simulink model "multi_UAV_simulation_model"  (R2023b)
settings: Solver=FixedStepAuto  StartTime=0  StopTime=end_time  FixedStep=0.01  RelTol=1e-3
values from neighbouring files (symbols this model uses):
  M_gamma = double(M_gamma)    [variable_system.m]
undefined symbols (not defined in the file or in its folder): AX_all, AY_all, F_dist, f_max, gamma0, J, J_xi, m, opt_angle_table_mat, tau_rotor, x0
libraries: slpidlib x4
settings Model: Creator=mochida  LastModifiedBy=tito
settings SolverCC: AlgebraicLoopSolver=TrustRegion
settings DataIOCC: SaveFormat=StructureWithTime  ReturnWorkspaceOutputs=off
settings OptimizationCC: BlockReduction=off  BufferReuse=off
settings DebuggingCC: AlgebraicLoopMsg=none  ArithmeticOperatorsInVariantConditions=warning
settings ModelReferenceCC: EnableRefExpFcnMdlSchedulingChecks=on
settings SFSimCC: SimUseLocalCustomCode=off  CustomCodeUndefinedFunction=UseInterfaceOnly
settings RTWCC: RTWUseLocalCustomCode=off  DLArmComputeVersion=19.05
settings ExplorerConfigSet: SimMechanicsOpenEditorOnUpdate=off

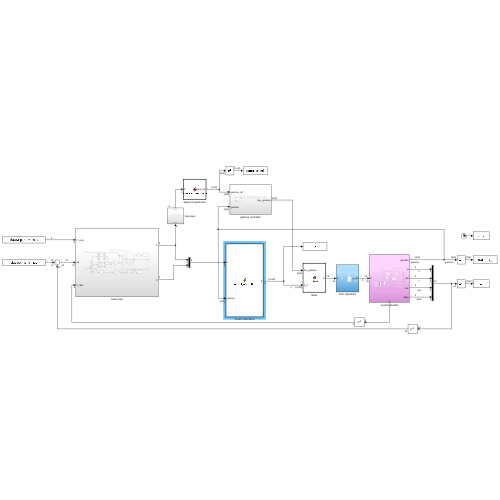
[thumbnail: Simulink's stored preview of the top-level diagram]
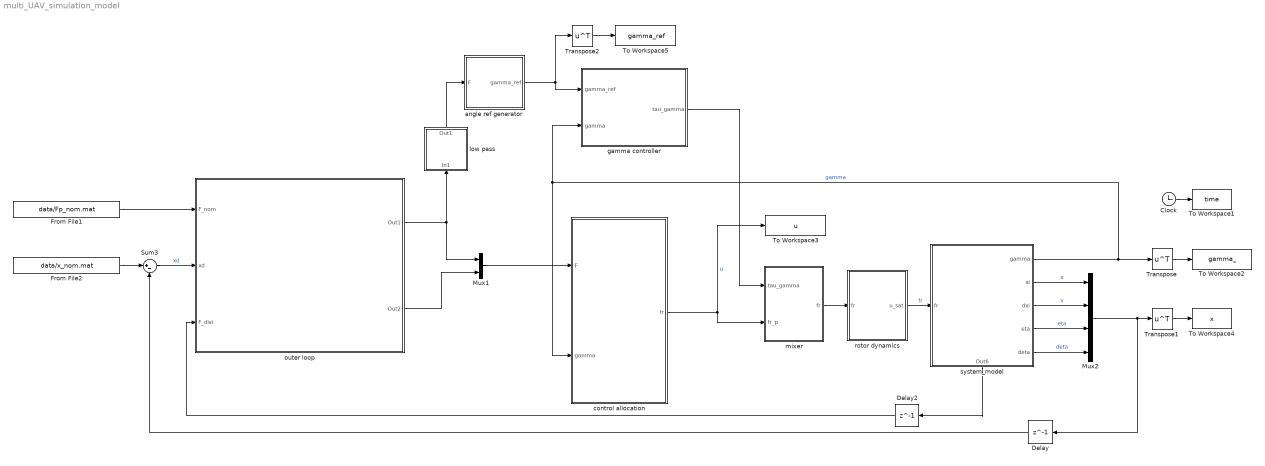
== system multi_UAV_simulation_model ==
  Clock : Clock
  Delay : Delay  DelayLength=1  InitialCondition=x0
  Delay2 : Delay  DelayLength=1  InitialCondition=zeros(3,1)
  From File1 : FromFile  FileName=data/Fp_nom.mat  SampleTime=0  ExtrapolationAfterLastDataPoint=Hold last value
  From File2 : FromFile  FileName=data/x_nom.mat  SampleTime=0  ExtrapolationAfterLastDataPoint=Hold last value
  Mux1 : Mux  Inputs=2
  Mux2 : Mux
  Sum3 : Sum  Inputs=|+-
  To Workspace1 : ToWorkspace  VariableName=time  SampleTime=-1
  To Workspace2 : ToWorkspace  VariableName=gamma_  SampleTime=-1
      settings: Save2DSignal=2-D array (concatenate along first dimension)
  To Workspace3 : ToWorkspace  VariableName=u  SampleTime=-1
  To Workspace4 : ToWorkspace  VariableName=x  SampleTime=-1
      settings: Save2DSignal=2-D array (concatenate along first dimension)
  To Workspace5 : ToWorkspace  VariableName=gamma_ref  SampleTime=-1
      settings: Save2DSignal=2-D array (concatenate along first dimension)
  Transpose : Math  Operator=transpose
  Transpose1 : Math  Operator=transpose
  Transpose2 : Math  Operator=transpose
  angle ref generator : MATLAB Function  TreatAsAtomicUnit=on
  control allocation : MATLAB Function  TreatAsAtomicUnit=on
  gamma controller : Subsystem
  low pass : Subsystem
  mixer : MATLAB Function  TreatAsAtomicUnit=on
  outer loop : Subsystem
  rotor dynamics : Subsystem
  system_model : Subsystem
      settings: PortSchema="{\"entries\":[{\"content\":{\"sides\":[{\"content\":{\"connectorIds\":[\"In1\"]},\"type\":\"ConnectorPlacement.EquallySpacedRectSide\",\"uuid\":\"254c1886-4b3f-4fd7-a815-da90215f9171\"},{\"content\":{\"connectorIds\":[\"Out1\",\"Out2\",\"Out3\",\"Out4\",\"Out5\"],\"side\":\"RIGHT\"},\"type\":\"ConnectorPlacement.EquallySpacedRectSide\",\"uuid\":\"0b427131-5008-4b05-bf64-69ca1b176e39\"},{\"content\":{\"side\":\"TOP\"},\"type\":\"ConnectorPlacement.EquallySpacedRectSide\",\"uuid\":\"ac393484-bc2a-4ae6-a0d7-f6f44710c509\"},{\"content\":{\"connectorIds\":[\"Out6\"],\"side\":\"BOTTOM\"},\"type\":\"ConnectorPlacement.EquallySpacedRectSide\",\"uuid\":\"d50d45f9-0e3b-4b3e-8f4a-1a82dc9ea554\"}]},\"type\":\"ConnectorPlacement.EquallySpacedConnector\",\"uuid\":\"c72c2ee8-503c-4769-877b-d1646d141d46\"}],\"packageUris\":[\"http://schema.mathworks.com/mf0/Connector/R2020b\"],\"version\":\"1.0\"}"
  wires:
  Clock/1 -> To Workspace1/1
  system_model/2(xi) -> Mux2/1  "x"
  system_model/3(dxi) -> Mux2/2  "v"
  system_model/4(eta) -> Mux2/3  "eta"
  system_model/5(deta) -> Mux2/4  "deta"
  rotor dynamics/1(u_sat) -> system_model/1(fr)  "fr"
  control allocation/1(fr) -> To Workspace3/1, mixer/2(fr_p)  "u"
  Delay/1 -> Sum3/2
  mixer/1(fr) -> rotor dynamics/1(fr)
  From File2/1 -> Sum3/1
  Mux2/1 -> Delay/1, Transpose1/1
  Transpose/1 -> To Workspace2/1
  Transpose1/1 -> To Workspace4/1
  system_model/1(gamma) -> gamma controller/2(gamma), control allocation/2(gamma), Transpose/1  "gamma"
  Mux1/1 -> control allocation/1(F)
  gamma controller/1(tau_gamma) -> mixer/1(tau_gamma)
  low pass/1(Out1) -> angle ref generator/1(F)
  angle ref generator/1(gamma_ref) -> Transpose2/1, gamma controller/1(gamma_ref)
  system_model/6(Out6) -> Delay2/1
  outer loop/1(Out1) -> low pass/1(In1), Mux1/1
  Sum3/1 -> outer loop/2(xd)  "xd"
  Delay2/1 -> outer loop/3(F_dist)
  outer loop/2(Out2) -> Mux1/2
  From File1/1 -> outer loop/1(F_nom)
  Transpose2/1 -> To Workspace5/1

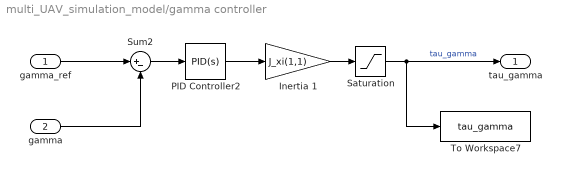
== system multi_UAV_simulation_model/gamma controller ==
  gamma_ref : Inport
  gamma : Inport  Port=2
  Inertia 1 : Gain  Gain=J_xi(1,1)
  PID Controller2 : slpidlib/PID Controller  Controller=PID  Form=Parallel  TimeDomain=Continuous-time  UseExternalTs=off  SampleTime=-1  IntegratorMethod=Forward Euler  FilterMethod=Forward Euler  ControllerParametersSource=internal  P=20  I=1  UseKiTs=off  D=5  N=209.794311620465  UseFilter=on  TunerSelectOption=Transfer Function Based (PID Tuner App)  InitialConditionSource=internal  InitialConditionForIntegrator=0  InitialConditionForFilter=0  DifferentiatorICPrevScaledInput=0  ExternalReset=none  TrackingMode=off  Kt=1  LimitOutput=off  SatLimitsSource=internal  UpperSaturationLimit=inf  LowerSaturationLimit=-inf  LinearizeAsGain=on  AntiWindupMode=none  Kb=1  LimitIntegrator=off  UpperIntegratorSaturationLimit=inf  LowerIntegratorSaturationLimit=-inf  POutMin=[]  POutMax=[]  IOutMin=[]  IOutMax=[]  DOutMin=[]  DOutMax=[]  NOutMin=[]  NOutMax=[]  SumOutMin=[]  SumOutMax=[]  SaturationOutMin=[]  SaturationOutMax=[]  PParamMin=[]  PParamMax=[]  IParamMin=[]  IParamMax=[]  DParamMin=[]  DParamMax=[]  NParamMin=[]  NParamMax=[]  KbParamMin=[]  KbParamMax=[]  KtParamMin=[]  KtParamMax=[]  KbOutMin=[]  KbOutMax=[]  KtOutMin=[]  KtOutMax=[]  IntegratorOutMin=[]  IntegratorOutMax=[]  FilterOutMin=[]  FilterOutMax=[]  SumI1OutMin=[]  SumI1OutMax=[]  SumI2OutMin=[]  SumI2OutMax=[]  SumI3OutMin=[]  SumI3OutMax=[]  SumI4OutMin=[]  SumI4OutMax=[]  SumDOutMin=[]  SumDOutMax=[]  DifferentiatorOutMin=[]  DifferentiatorOutMax=[]  FilterDiffOutCoefMin=[]  FilterDiffOutCoefMax=[]  ReciprocalOutMin=[]  ReciprocalOutMax=[]  SumDenOutMin=[]  SumDenOutMax=[]  SumNumOutMin=[]  SumNumOutMax=[]  DivideOutMin=[]  DivideOutMax=[]  UdiffTsProdOutMin=[]  UdiffTsProdOutMax=[]  NTsProdOutMin=[]  NTsProdOutMax=[]  UintegralTsProdOutMin=[]  UintegralTsProdOutMax=[]  UngainTsProdOutMin=[]  UngainTsProdOutMax=[]  ClampingZeroOutDataTypeStr=Inherit: Inherit via back propagation  ClampingZeroOutMin=[]  ClampingZeroOutMax=[]  FilterDenConstantOutDataTypeStr=Inherit: Inherit via back propagation  FilterDenConstantOutMin=[]  FilterDenConstantOutMax=[]  PCopyOutDataTypeStr=Inherit: Inherit via back propagation  PCopyOutMin=[]  PCopyOutMax=[]  NCopyOutDataTypeStr=Inherit: Inherit via back propagation  NCopyOutMin=[]  NCopyOutMax=[]  IntegratorContinuousStateAttributes=''  IntegratorStateMustResolveToSignalObject=off  IntegratorRTWStateStorageClass=Auto  FilterContinuousStateAttributes=''  FilterStateMustResolveToSignalObject=off  FilterRTWStateStorageClass=Auto  ParallelPVariant=InternalParameters  IdealPVariant=Disabled  IVariant=InternalParameters  DVariant=InternalParameters  IntegratorVariant=Continuous  SatVariant=Disabled  AWVariant=Passthrough  PCopyVariant=Disabled  TRVariant=Disabled  FdbkBlocksVariant=Forward  IdealPFdbkVariant=Disabled  SatFdbkVariant=Disabled  DerivativeFilterVariant=ContFilter  NVariant=InternalParameters  NCopyVariant=Disabled  FilterICVariant=InternalICsFilter  IntegratorICVariant=InternalICs  ExternalResetVariant=Disabled  TRSumVariant=Passthrough  SumFdbkVariant=Disabled  SumVariant=Sum_PID  TsampFilterVariant=InternalTs  TsampNgainVariant=Passthrough  TsampIntegralVariant=Disabled_SignalSpec  ExternalSaturationOutDataTypeStr=Inherit: Same as second input
  Saturation : Saturate  UpperLimit=0.03  LowerLimit=-0.03
  Sum2 : Sum  Inputs=|+-
  To Workspace7 : ToWorkspace  VariableName=tau_gamma  SaveFormat=Timeseries  SampleTime=-1
  tau_gamma : Outport
  wires:
  Inertia 1/1 -> Saturation/1
  Sum2/1 -> PID Controller2/1
  Saturation/1 -> tau_gamma/1, To Workspace7/1  "tau_gamma"
  PID Controller2/1 -> Inertia 1/1
  gamma/1 -> Sum2/2
  gamma_ref/1 -> Sum2/1

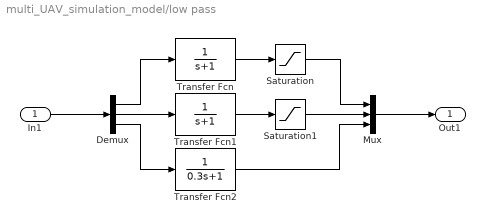
== system multi_UAV_simulation_model/low pass ==
  In1 : Inport
  Demux : Demux  Outputs=3
  Mux : Mux  Inputs=3
  Saturation : Saturate  UpperLimit=1  LowerLimit=-1
  Saturation1 : Saturate  UpperLimit=1  LowerLimit=-1
  Transfer Fcn : TransferFcn  Denominator=[1 1]
  Transfer Fcn1 : TransferFcn  Denominator=[1 1]
  Transfer Fcn2 : TransferFcn  Denominator=[0.3 1]
  Out1 : Outport
  wires:
  In1/1 -> Demux/1
  Demux/3 -> Transfer Fcn2/1
  Demux/2 -> Transfer Fcn1/1
  Mux/1 -> Out1/1
  Transfer Fcn2/1 -> Mux/3
  Transfer Fcn1/1 -> Saturation1/1
  Transfer Fcn/1 -> Saturation/1
  Demux/1 -> Transfer Fcn/1
  Saturation/1 -> Mux/1
  Saturation1/1 -> Mux/2

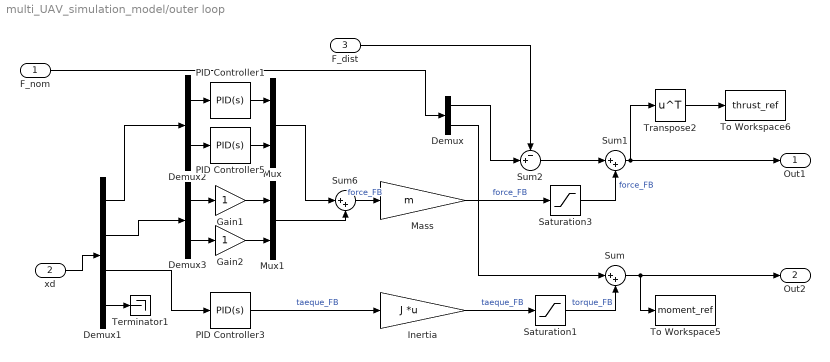
== system multi_UAV_simulation_model/outer loop ==
  F_nom : Inport
  xd : Inport  Port=2
  F_dist : Inport  Port=3
  Demux : Demux  Outputs=2
  Demux1 : Demux  Outputs=[3 3 3 3]
  Demux2 : Demux  Outputs=[2 1]
  Demux3 : Demux  Outputs=[2 1]
  Gain1 : Gain
  Gain2 : Gain
  "Inertia " : Gain  Gain=J  Multiplication=Matrix(K*u) (u vector)
  Mass : Gain  Gain=m
  Mux : Mux  Inputs=2
  Mux1 : Mux  Inputs=2
  PID Controller1 : slpidlib/PID Controller  Controller=PID  Form=Parallel  TimeDomain=Continuous-time  UseExternalTs=off  SampleTime=-1  IntegratorMethod=Forward Euler  FilterMethod=Forward Euler  ControllerParametersSource=internal  P=1  I=1/10  UseKiTs=off  D=0  N=10.9079405084324  UseFilter=on  TunerSelectOption=Transfer Function Based (PID Tuner App)  InitialConditionSource=internal  InitialConditionForIntegrator=0  InitialConditionForFilter=0  DifferentiatorICPrevScaledInput=0  ExternalReset=none  TrackingMode=off  Kt=1  LimitOutput=off  SatLimitsSource=internal  UpperSaturationLimit=inf  LowerSaturationLimit=-inf  LinearizeAsGain=on  AntiWindupMode=none  Kb=1  LimitIntegrator=off  UpperIntegratorSaturationLimit=inf  LowerIntegratorSaturationLimit=-inf  POutMin=[]  POutMax=[]  IOutMin=[]  IOutMax=[]  DOutMin=[]  DOutMax=[]  NOutMin=[]  NOutMax=[]  SumOutMin=[]  SumOutMax=[]  SaturationOutMin=[]  SaturationOutMax=[]  PParamMin=[]  PParamMax=[]  IParamMin=[]  IParamMax=[]  DParamMin=[]  DParamMax=[]  NParamMin=[]  NParamMax=[]  KbParamMin=[]  KbParamMax=[]  KtParamMin=[]  KtParamMax=[]  KbOutMin=[]  KbOutMax=[]  KtOutMin=[]  KtOutMax=[]  IntegratorOutMin=[]  IntegratorOutMax=[]  FilterOutMin=[]  FilterOutMax=[]  SumI1OutMin=[]  SumI1OutMax=[]  SumI2OutMin=[]  SumI2OutMax=[]  SumI3OutMin=[]  SumI3OutMax=[]  SumI4OutMin=[]  SumI4OutMax=[]  SumDOutMin=[]  SumDOutMax=[]  DifferentiatorOutMin=[]  DifferentiatorOutMax=[]  FilterDiffOutCoefMin=[]  FilterDiffOutCoefMax=[]  ReciprocalOutMin=[]  ReciprocalOutMax=[]  SumDenOutMin=[]  SumDenOutMax=[]  SumNumOutMin=[]  SumNumOutMax=[]  DivideOutMin=[]  DivideOutMax=[]  UdiffTsProdOutMin=[]  UdiffTsProdOutMax=[]  NTsProdOutMin=[]  NTsProdOutMax=[]  UintegralTsProdOutMin=[]  UintegralTsProdOutMax=[]  UngainTsProdOutMin=[]  UngainTsProdOutMax=[]  ClampingZeroOutDataTypeStr=Inherit: Inherit via back propagation  ClampingZeroOutMin=[]  ClampingZeroOutMax=[]  FilterDenConstantOutDataTypeStr=Inherit: Inherit via back propagation  FilterDenConstantOutMin=[]  FilterDenConstantOutMax=[]  PCopyOutDataTypeStr=Inherit: Inherit via back propagation  PCopyOutMin=[]  PCopyOutMax=[]  NCopyOutDataTypeStr=Inherit: Inherit via back propagation  NCopyOutMin=[]  NCopyOutMax=[]  IntegratorContinuousStateAttributes=''  IntegratorStateMustResolveToSignalObject=off  IntegratorRTWStateStorageClass=Auto  FilterContinuousStateAttributes=''  FilterStateMustResolveToSignalObject=off  FilterRTWStateStorageClass=Auto  ParallelPVariant=InternalParameters  IdealPVariant=Disabled  IVariant=InternalParameters  DVariant=InternalParameters  IntegratorVariant=Continuous  SatVariant=Disabled  AWVariant=Passthrough  PCopyVariant=Disabled  TRVariant=Disabled  FdbkBlocksVariant=Forward  IdealPFdbkVariant=Disabled  SatFdbkVariant=Disabled  DerivativeFilterVariant=ContFilter  NVariant=InternalParameters  NCopyVariant=Disabled  FilterICVariant=InternalICsFilter  IntegratorICVariant=InternalICs  ExternalResetVariant=Disabled  TRSumVariant=Passthrough  SumFdbkVariant=Disabled  SumVariant=Sum_PID  TsampFilterVariant=InternalTs  TsampNgainVariant=Passthrough  TsampIntegralVariant=Disabled_SignalSpec  ExternalSaturationOutDataTypeStr=Inherit: Same as second input
  PID Controller3 : slpidlib/PID Controller  Controller=PID  Form=Parallel  TimeDomain=Continuous-time  UseExternalTs=off  SampleTime=-1  IntegratorMethod=Forward Euler  FilterMethod=Forward Euler  ControllerParametersSource=internal  P=10  I=10  UseKiTs=off  D=10  N=10.9079405084324  UseFilter=on  TunerSelectOption=Transfer Function Based (PID Tuner App)  InitialConditionSource=internal  InitialConditionForIntegrator=0  InitialConditionForFilter=0  DifferentiatorICPrevScaledInput=0  ExternalReset=none  TrackingMode=off  Kt=1  LimitOutput=off  SatLimitsSource=internal  UpperSaturationLimit=inf  LowerSaturationLimit=-inf  LinearizeAsGain=on  AntiWindupMode=none  Kb=1  LimitIntegrator=off  UpperIntegratorSaturationLimit=inf  LowerIntegratorSaturationLimit=-inf  POutMin=[]  POutMax=[]  IOutMin=[]  IOutMax=[]  DOutMin=[]  DOutMax=[]  NOutMin=[]  NOutMax=[]  SumOutMin=[]  SumOutMax=[]  SaturationOutMin=[]  SaturationOutMax=[]  PParamMin=[]  PParamMax=[]  IParamMin=[]  IParamMax=[]  DParamMin=[]  DParamMax=[]  NParamMin=[]  NParamMax=[]  KbParamMin=[]  KbParamMax=[]  KtParamMin=[]  KtParamMax=[]  KbOutMin=[]  KbOutMax=[]  KtOutMin=[]  KtOutMax=[]  IntegratorOutMin=[]  IntegratorOutMax=[]  FilterOutMin=[]  FilterOutMax=[]  SumI1OutMin=[]  SumI1OutMax=[]  SumI2OutMin=[]  SumI2OutMax=[]  SumI3OutMin=[]  SumI3OutMax=[]  SumI4OutMin=[]  SumI4OutMax=[]  SumDOutMin=[]  SumDOutMax=[]  DifferentiatorOutMin=[]  DifferentiatorOutMax=[]  FilterDiffOutCoefMin=[]  FilterDiffOutCoefMax=[]  ReciprocalOutMin=[]  ReciprocalOutMax=[]  SumDenOutMin=[]  SumDenOutMax=[]  SumNumOutMin=[]  SumNumOutMax=[]  DivideOutMin=[]  DivideOutMax=[]  UdiffTsProdOutMin=[]  UdiffTsProdOutMax=[]  NTsProdOutMin=[]  NTsProdOutMax=[]  UintegralTsProdOutMin=[]  UintegralTsProdOutMax=[]  UngainTsProdOutMin=[]  UngainTsProdOutMax=[]  ClampingZeroOutDataTypeStr=Inherit: Inherit via back propagation  ClampingZeroOutMin=[]  ClampingZeroOutMax=[]  FilterDenConstantOutDataTypeStr=Inherit: Inherit via back propagation  FilterDenConstantOutMin=[]  FilterDenConstantOutMax=[]  PCopyOutDataTypeStr=Inherit: Inherit via back propagation  PCopyOutMin=[]  PCopyOutMax=[]  NCopyOutDataTypeStr=Inherit: Inherit via back propagation  NCopyOutMin=[]  NCopyOutMax=[]  IntegratorContinuousStateAttributes=''  IntegratorStateMustResolveToSignalObject=off  IntegratorRTWStateStorageClass=Auto  FilterContinuousStateAttributes=''  FilterStateMustResolveToSignalObject=off  FilterRTWStateStorageClass=Auto  ParallelPVariant=InternalParameters  IdealPVariant=Disabled  IVariant=InternalParameters  DVariant=InternalParameters  IntegratorVariant=Continuous  SatVariant=Disabled  AWVariant=Passthrough  PCopyVariant=Disabled  TRVariant=Disabled  FdbkBlocksVariant=Forward  IdealPFdbkVariant=Disabled  SatFdbkVariant=Disabled  DerivativeFilterVariant=ContFilter  NVariant=InternalParameters  NCopyVariant=Disabled  FilterICVariant=InternalICsFilter  IntegratorICVariant=InternalICs  ExternalResetVariant=Disabled  TRSumVariant=Passthrough  SumFdbkVariant=Disabled  SumVariant=Sum_PID  TsampFilterVariant=InternalTs  TsampNgainVariant=Passthrough  TsampIntegralVariant=Disabled_SignalSpec  ExternalSaturationOutDataTypeStr=Inherit: Same as second input
  PID Controller5 : slpidlib/PID Controller  Controller=PID  Form=Parallel  TimeDomain=Continuous-time  UseExternalTs=off  SampleTime=-1  IntegratorMethod=Forward Euler  FilterMethod=Forward Euler  ControllerParametersSource=internal  P=1  I=1/10  UseKiTs=off  D=0  N=10.9079405084324  UseFilter=on  TunerSelectOption=Transfer Function Based (PID Tuner App)  InitialConditionSource=internal  InitialConditionForIntegrator=0  InitialConditionForFilter=0  DifferentiatorICPrevScaledInput=0  ExternalReset=none  TrackingMode=off  Kt=1  LimitOutput=off  SatLimitsSource=internal  UpperSaturationLimit=inf  LowerSaturationLimit=-inf  LinearizeAsGain=on  AntiWindupMode=none  Kb=1  LimitIntegrator=off  UpperIntegratorSaturationLimit=inf  LowerIntegratorSaturationLimit=-inf  POutMin=[]  POutMax=[]  IOutMin=[]  IOutMax=[]  DOutMin=[]  DOutMax=[]  NOutMin=[]  NOutMax=[]  SumOutMin=[]  SumOutMax=[]  SaturationOutMin=[]  SaturationOutMax=[]  PParamMin=[]  PParamMax=[]  IParamMin=[]  IParamMax=[]  DParamMin=[]  DParamMax=[]  NParamMin=[]  NParamMax=[]  KbParamMin=[]  KbParamMax=[]  KtParamMin=[]  KtParamMax=[]  KbOutMin=[]  KbOutMax=[]  KtOutMin=[]  KtOutMax=[]  IntegratorOutMin=[]  IntegratorOutMax=[]  FilterOutMin=[]  FilterOutMax=[]  SumI1OutMin=[]  SumI1OutMax=[]  SumI2OutMin=[]  SumI2OutMax=[]  SumI3OutMin=[]  SumI3OutMax=[]  SumI4OutMin=[]  SumI4OutMax=[]  SumDOutMin=[]  SumDOutMax=[]  DifferentiatorOutMin=[]  DifferentiatorOutMax=[]  FilterDiffOutCoefMin=[]  FilterDiffOutCoefMax=[]  ReciprocalOutMin=[]  ReciprocalOutMax=[]  SumDenOutMin=[]  SumDenOutMax=[]  SumNumOutMin=[]  SumNumOutMax=[]  DivideOutMin=[]  DivideOutMax=[]  UdiffTsProdOutMin=[]  UdiffTsProdOutMax=[]  NTsProdOutMin=[]  NTsProdOutMax=[]  UintegralTsProdOutMin=[]  UintegralTsProdOutMax=[]  UngainTsProdOutMin=[]  UngainTsProdOutMax=[]  ClampingZeroOutDataTypeStr=Inherit: Inherit via back propagation  ClampingZeroOutMin=[]  ClampingZeroOutMax=[]  FilterDenConstantOutDataTypeStr=Inherit: Inherit via back propagation  FilterDenConstantOutMin=[]  FilterDenConstantOutMax=[]  PCopyOutDataTypeStr=Inherit: Inherit via back propagation  PCopyOutMin=[]  PCopyOutMax=[]  NCopyOutDataTypeStr=Inherit: Inherit via back propagation  NCopyOutMin=[]  NCopyOutMax=[]  IntegratorContinuousStateAttributes=''  IntegratorStateMustResolveToSignalObject=off  IntegratorRTWStateStorageClass=Auto  FilterContinuousStateAttributes=''  FilterStateMustResolveToSignalObject=off  FilterRTWStateStorageClass=Auto  ParallelPVariant=InternalParameters  IdealPVariant=Disabled  IVariant=InternalParameters  DVariant=InternalParameters  IntegratorVariant=Continuous  SatVariant=Disabled  AWVariant=Passthrough  PCopyVariant=Disabled  TRVariant=Disabled  FdbkBlocksVariant=Forward  IdealPFdbkVariant=Disabled  SatFdbkVariant=Disabled  DerivativeFilterVariant=ContFilter  NVariant=InternalParameters  NCopyVariant=Disabled  FilterICVariant=InternalICsFilter  IntegratorICVariant=InternalICs  ExternalResetVariant=Disabled  TRSumVariant=Passthrough  SumFdbkVariant=Disabled  SumVariant=Sum_PID  TsampFilterVariant=InternalTs  TsampNgainVariant=Passthrough  TsampIntegralVariant=Disabled_SignalSpec  ExternalSaturationOutDataTypeStr=Inherit: Same as second input
  Saturation1 : Saturate  UpperLimit=0.1  LowerLimit=-0.1
  Saturation3 : Saturate  UpperLimit=1  LowerLimit=-1
  Sum : Sum  Inputs=|++
  Sum1 : Sum  Inputs=|++
  Sum2 : Sum  Inputs=-+|
  Sum6 : Sum  Inputs=|++
  Terminator1 : Terminator
  To Workspace5 : ToWorkspace  VariableName=moment_ref  SampleTime=-1
  To Workspace6 : ToWorkspace  VariableName=thrust_ref  SampleTime=-1
      settings: Save2DSignal=2-D array (concatenate along first dimension)
  Transpose2 : Math  Operator=transpose
  Out1 : Outport
  Out2 : Outport  Port=2
  wires:
  Mass/1 -> Saturation3/1  "force_FB"
  Demux1/4 -> Terminator1/1
  PID Controller3/1 -> "Inertia "/1  "taeque_FB"
  F_nom/1 -> Demux/1
  PID Controller5/1 -> Mux/2
  Demux1/1 -> Demux2/1
  xd/1 -> Demux1/1
  Sum1/1 -> Out1/1, Transpose2/1
  Sum2/1 -> Sum1/1
  Sum/1 -> Out2/1, To Workspace5/1
  Sum6/1 -> Mass/1  "force_FB"
  Saturation3/1 -> Sum1/2  "force_FB"
  "Inertia "/1 -> Saturation1/1  "taeque_FB"
  Demux/2 -> Sum/1
  Transpose2/1 -> To Workspace6/1
  F_dist/1 -> Sum2/1
  Demux/1 -> Sum2/2
  Demux1/3 -> PID Controller3/1
  Demux1/2 -> Demux3/1
  Saturation1/1 -> Sum/2  "torque_FB"
  Gain1/1 -> Mux1/1
  Demux2/2 -> PID Controller5/1
  Demux2/1 -> PID Controller1/1
  PID Controller1/1 -> Mux/1
  Mux/1 -> Sum6/1
  Demux3/1 -> Gain1/1
  Demux3/2 -> Gain2/1
  Gain2/1 -> Mux1/2
  Mux1/1 -> Sum6/2

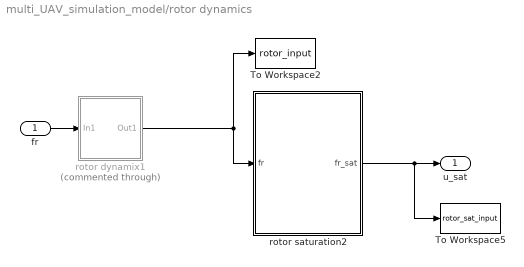
== system multi_UAV_simulation_model/rotor dynamics ==
  fr : Inport
  To Workspace2 : ToWorkspace  VariableName=rotor_input  SampleTime=-1
  To Workspace5 : ToWorkspace  VariableName=rotor_sat_input  SampleTime=-1
  rotor dynamix1 : Subsystem  Commented=through
  rotor saturation2 : MATLAB Function  TreatAsAtomicUnit=on
  u_sat : Outport
  wires:
  fr/1 -> rotor dynamix1/1(In1)
  rotor saturation2/1(fr_sat) -> To Workspace5/1, u_sat/1
  rotor dynamix1/1(Out1) -> To Workspace2/1, rotor saturation2/1(fr)

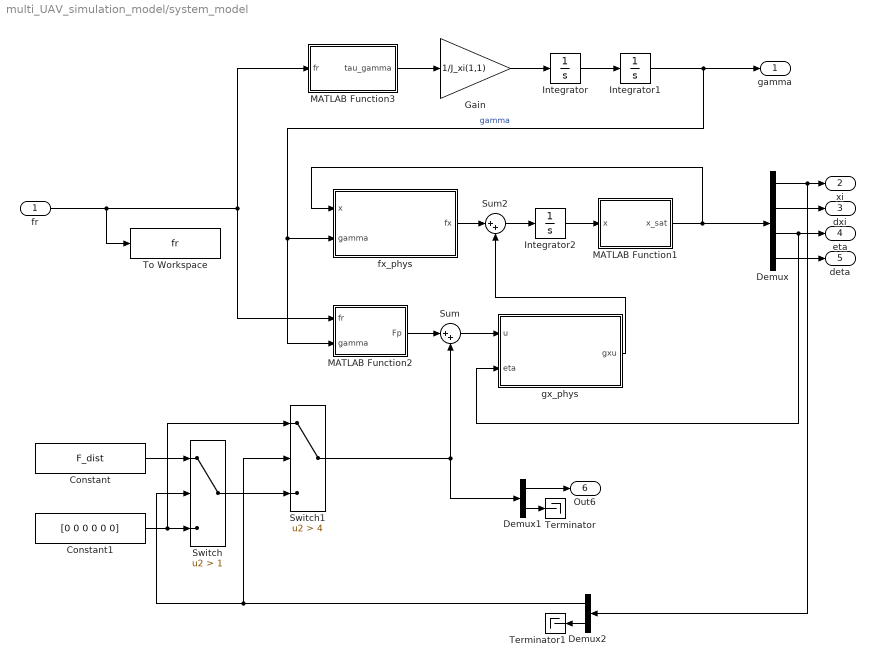
== system multi_UAV_simulation_model/system_model ==
  fr : Inport
  Constant : Constant  Value=F_dist
  Constant1 : Constant  Value=[0 0 0 0 0 0]
  Demux : Demux  Outputs=[3 3 3 3]
  Demux1 : Demux  Outputs=[3 3]
  Demux2 : Demux  Outputs=[1 2]
  Gain : Gain  Gain=1/J_xi(1,1)
  Integrator : Integrator  InitialCondition=zeros(4,1)
  Integrator1 : Integrator  InitialCondition=gamma0
  Integrator2 : Integrator  InitialCondition=x0
  MATLAB Function1 : MATLAB Function  TreatAsAtomicUnit=on
  MATLAB Function2 : MATLAB Function  TreatAsAtomicUnit=on
  MATLAB Function3 : MATLAB Function  TreatAsAtomicUnit=on
  Sum : Sum  Inputs=|++
  Sum2 : Sum  Inputs=|++
  Switch : Switch  Criteria=u2 > Threshold  Threshold=1  SaturateOnIntegerOverflow=off  InputSameDT=off
  Switch1 : Switch  Criteria=u2 > Threshold  Threshold=4  SaturateOnIntegerOverflow=off  InputSameDT=off
  Terminator : Terminator
  Terminator1 : Terminator
  To Workspace : ToWorkspace  VariableName=fr  SampleTime=-1
  fx_phys : MATLAB Function  TreatAsAtomicUnit=on
  gx_phys : MATLAB Function  TreatAsAtomicUnit=on
  gamma : Outport  VectorParamsAs1DForOutWhenUnconnected=off
  xi : Outport  Port=2  VectorParamsAs1DForOutWhenUnconnected=off
  dxi : Outport  Port=3  VectorParamsAs1DForOutWhenUnconnected=off
  eta : Outport  Port=4  VectorParamsAs1DForOutWhenUnconnected=off
  deta : Outport  Port=5  VectorParamsAs1DForOutWhenUnconnected=off
  Out6 : Outport  Port=6
  wires:
  fx_phys/1(fx) -> Sum2/1
  Demux/3 -> eta/1, gx_phys/2(eta)
  Demux/4 -> deta/1
  Demux/1 -> Demux2/1, xi/1
  MATLAB Function1/1(x_sat) -> fx_phys/1(x), Demux/1
  Demux/2 -> dxi/1
  gx_phys/1(gxu) -> Sum2/2
  Integrator2/1 -> MATLAB Function1/1(x)
  Sum2/1 -> Integrator2/1
  fr/1 -> MATLAB Function3/1(fr), MATLAB Function2/1(fr), To Workspace/1
  MATLAB Function3/1(tau_gamma) -> Gain/1
  Integrator/1 -> Integrator1/1
  Integrator1/1 -> MATLAB Function2/2(gamma), fx_phys/2(gamma), gamma/1  "gamma"
  Gain/1 -> Integrator/1
  MATLAB Function2/1(Fp) -> Sum/1
  Constant/1 -> Switch/1
  Sum/1 -> gx_phys/1(u)
  Switch/1 -> Switch1/3
  Constant1/1 -> Switch1/1, Switch/3
  Switch1/1 -> Demux1/1, Sum/2
  Demux1/1 -> Out6/1
  Demux1/2 -> Terminator/1
  Demux2/2 -> Terminator1/1
  Demux2/1 -> Switch1/2, Switch/2

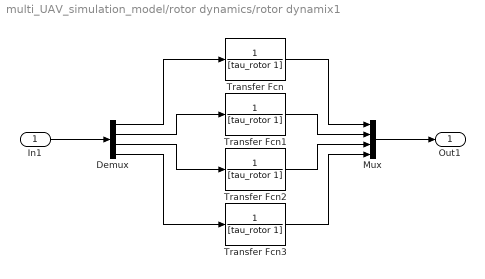
== system multi_UAV_simulation_model/rotor dynamics/rotor dynamix1 ==
  In1 : Inport
  Demux : Demux
  Mux : Mux
  Transfer Fcn{,1..3} (4 alike) : TransferFcn  Denominator=[tau_rotor 1]
  Out1 : Outport
  wires:
  In1/1 -> Demux/1
  Demux/4 -> Transfer Fcn3/1
  Demux/3 -> Transfer Fcn2/1
  Demux/2 -> Transfer Fcn1/1
  Mux/1 -> Out1/1
  Transfer Fcn3/1 -> Mux/4
  Transfer Fcn2/1 -> Mux/3
  Transfer Fcn1/1 -> Mux/2
  Transfer Fcn/1 -> Mux/1
  Demux/1 -> Transfer Fcn/1

== matlab function multi_UAV_simulation_model/mixer ==
  data: tau_gamma input; fr_p input; fr output; M_gamma parameter
function fr = mixer(tau_gamma,fr_p, M_gamma)
    
    fr_gamma = M_gamma \ tau_gamma;

    fr = fr_p' + fr_gamma;

== matlab function multi_UAV_simulation_model/system_model/fx_phys ==
  data: x input; fx output; gamma input
function fx=fx_phys(x,gamma)

%this function generated in "variable_system.m"
fx=fx_fun(x,gamma);

== matlab function multi_UAV_simulation_model/system_model/MATLAB Function2 ==
  data: fr input; Fp output; gamma input
function Fp = fcn(fr, gamma)

Fp = M_ftau_fun(gamma')*fr;

== matlab function multi_UAV_simulation_model/angle ref generator ==
  data: F input; gamma_ref output; opt_angle_table_mat parameter; AX_all parameter; AY_all parameter
function gamma_ref = generate_gamma_ref(F, opt_angle_table_mat, AX_all, AY_all)

gamma_ref = zeros(4,1);
for i=1:4
    opt_angle_tmp = reshape(opt_angle_table_mat(i,:,:),size(AX_all));
    gamma_ref(i) = interp2(AX_all, AY_all, opt_angle_tmp', F(1), F(2),'cubic');
end

== matlab function multi_UAV_simulation_model/control allocation ==
  data: F input; fr output; gamma input; f_max parameter; M_gamma parameter
function fr= control_allocation(F, gamma, f_max, M_gamma)

coder.extrinsic('lsqminnorm');
coder.extrinsic('linprog');

N = length(gamma);

% f_mid = norm(F(1:3))/(4*N);
f_mid = 0;

f = [zeros(1,4*N), 1, -1];
A = [eye(4*N), -ones(4*N,1), zeros(4*N,1);
     -eye(4*N), zeros(4*N,1), ones(4*N,1);
     zeros(1,4*N), 0, -1];
b = [f_mid*ones(4*N,1); -f_mid*ones(4*N,1); 0];

M_ftau = M_ftau_fun(gamma');

Aeq = [M_ftau, zeros(6,2);
       M_gamma, zeros(N,2)];
beq = [F; zeros(N,1)];

lb = [0.1*ones(1,4*N+2)];
ub = [f_max*ones(1,4*N+2)];

flag = 0;
fr = zeros(1, 4*N);
[fr_opt, ~, flag, ~] = linprog(f,A,b,Aeq,beq,lb,ub);

% if liner problem has no optimizer
if flag==-2
    M_ftau = M_ftau_fun(gamma');    
    fr(1:4*N) = M_ftau\F;
else
    fr(1:4*N) = fr_opt(1:4*N)';
end

end

% N = length(gamma);
% 
% f = [zeros(1,4*N), 1];
% A = [-eye(4*N), 0.1*ones(4*N,1);
%      eye(4*N), -f_max*ones(4*N,1);
%      zeros(1,4*N), -1];
% b = zeros(8*N+1,1);
% if is_fix
%     Aeq = [Mp_fun(gamma), zeros(6,1)];
%     beq = F;
% else
%     Aeq = [Mp_fun(gamma), zeros(6,1);
%                   M_gamma, zeros(N,1)];
%     beq = [F; zeros(N,1)];
% end
% 
% flag = 0;
% fr = zeros(1, 4*N);
% [fr_opt, ~, flag, ~] = linprog(f,A,b,Aeq,beq,[],[]);
% 
% % if liner problem has no optimizer
% if flag==-2
%     Mp = Mp_fun(gamma);    
%     fr(1:4*N) = Mp\F;
% else
%     fr(1:4*N) = fr_opt(1:4*N)';
% end
% 
% end

== matlab function multi_UAV_simulation_model/system_model/MATLAB Function3 ==
  data: fr input; tau_gamma output; M_gamma parameter
function tau_gamma = fcn(fr, M_gamma)

    tau_gamma = M_gamma * fr;

== matlab function multi_UAV_simulation_model/system_model/gx_phys ==
  data: u input; gxu output; eta input
function gxu=gx_phys(u,eta)
%this function generated in "variable_system.m"

gxu=gx_fun(eta)*u;

== matlab function multi_UAV_simulation_model/system_model/MATLAB Function1 ==
  data: x input; x_sat output
function x_sat = z_satulation(x)

    x_sat = x;
    if x(3) < 0.1
        x_sat(3)=0.1;
        % if x(6)<0
        %     x_sat(6)=0;
        % end
    end
    
end

== matlab function multi_UAV_simulation_model/rotor dynamics/rotor saturation2 ==
  data: fr input; fr_sat output; f_max parameter
function fr_sat = input_saturation(fr,f_max)

fr_sat = zeros(size(fr));

fr_sat = max(fr,zeros(size(fr)));
fr_sat = min(fr_sat,f_max*ones(size(fr)));
